simulink library "MyPMSMLibrary"  (R2025b)
settings: Solver=VariableStepAuto  StartTime=0.0  StopTime=10.0  RelTol=1e-3
settings Model: Creator=jff_1  LastModifiedBy=jff_1
settings ModelReferenceCC: EnableRefExpFcnMdlSchedulingChecks=on
settings RTWCC: GPUComputeCapability=3.5

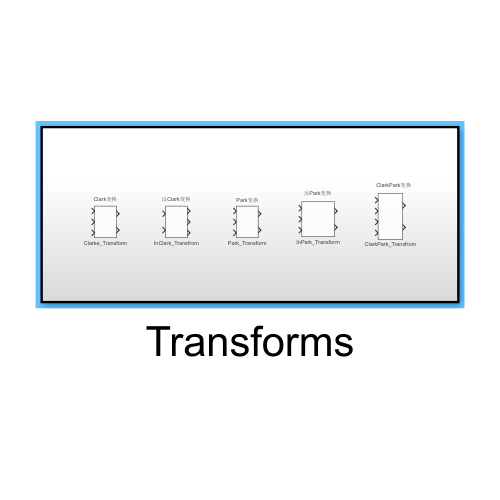
[thumbnail: Simulink's stored preview of the top-level diagram]
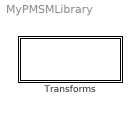
== system MyPMSMLibrary ==
  Transforms : Subsystem

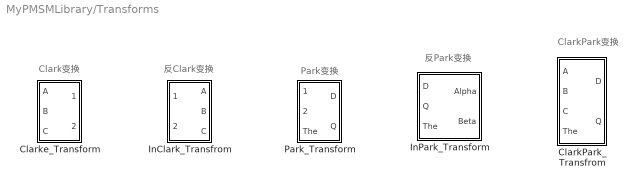
== system MyPMSMLibrary/Transforms ==
  note: 反Clark变换
  note: Clark变换
  note: Park变换
  note: 反Park变换
  note: ClarkPark变换
  ClarkPark_Transfrom : Subsystem
      mask help:
      | 将三相静止坐标系的 A、B、C 量通过同步旋转角 The(θ) 变换到同步旋转坐标系 d、q。
      | 本模块采用 2/3 幅值不变（amplitude-invariant）系数，常用于电机矢量控制中的电流/电压坐标变换。
      mask Help:
      | 【功能】
      | 把三相静止量 (A,B,C) 变换为同步旋转坐标系的 (d,q)，角度由 The(θ) 提供。
      | 
      | 【输入端口】
      | 
      | A：A 相量（电流/电压等）
      | 
      | B：B 相量
      | 
      | C：C 相量
      | 
      | The：同步旋转角 θ（单位：rad，弧度）
      | 
      | 【输出端口】
      | 
      | D：d 轴分量
      | 
      | Q：q 轴分量
      | 
      | 【计算关系（与模块内部 Fcn 一致）】
      | D = ( Acos(The) + Bcos(The - 2/3pi) + Ccos(The + 2/3pi) ) * 2/3
      | Q = -( Asin(The) + Bsin(The - 2/3pi) + Csin(The + 2/3pi) ) * 2/3
      | 
      | 【说明与注意】
      | 
      | The 必须使用弧度制；若你手里是角度制(°)，请先转换：The = The_deg*pi/180。
      | 
      | 该实现等价于“Clarke(abc→αβ) + Park(αβ→dq)”的组合写法，只是把两步合成到一起。
      | 
      | 若输入三相为对称系统（A+B+C=0），该变换结果最稳定；若含零序分量，本模块未单独输出零序。
      | 
      | 【快速自检建议】
      | 
      | 令 The = 0：此时 D 与 A 的相关性最大，Q 主要由 B/C 组合决定。
      | 
      | 令三相为对称正弦并随 The 同步旋转：理想情况下 d 为常值、q 约为 0（或相反，取决于相位定义）。
      mask DialogControl ParameterGroupVar Prompt: 参数
      mask Display:
      | % 输入端口
      | port_label('input',1,'A');
      | port_label('input',2,'B');
      | port_label('input',3,'C');
      | port_label('input',4,'The');
      | 
      | % 输出端口
      | port_label('output',1,'D');
      | port_label('output',2,'Q');
  Clarke_Transform : Subsystem
      mask help:
      | Clarke 坐标变换（abc → αβ）
      |
      | 采用幅值不变形式（2/3 系数）
      | 适用于三相对称、无零序分量的系统
      mask Help: 现代永磁同步电机控制原理及MATLAB仿真P5
      mask DialogControl ParameterGroupVar Prompt: 参数
      mask Display:
      | % 输入端口标签（1~3）
      | port_label('input',1,'A');
      | port_label('input',2,'B');
      | port_label('input',3,'C');
      | 
      | % 输出端口标签（1~2）
      | port_label('output',1,'Alpha');
      | port_label('output',2,'Beta');
  InClark_Transfrom : Subsystem
      mask help:
      | 反Clark坐标变换（αβ → abc）
      |
      | 采用幅值不变形式（2/3 系数）
      | 适用于三相对称、无零序分量的系统
      mask Help: 现代永磁同步电机控制原理及MATLAB仿真P6
      mask DialogControl ParameterGroupVar Prompt: 参数
      mask Display:
      | % 输入端口标签（1~3）
      | port_label('input',1,'Alpha');
      | port_label('input',2,'Beta');
      | 
      | % 输出端口标签（1~2）
      | port_label('output',1,'A');
      | port_label('output',2,'B');
      | port_label('output',3,'C');
  InPark_Transform : Subsystem
      mask help:
      | 反 Park 变换用于将同步旋转坐标系 d–q 中的变量变换回静止坐标系 α–β。
      | 该变换是 Park 变换的逆过程，广泛应用于 PMSM 矢量控制（FOC）中，
      | 用于将 dq 坐标系下的电流或电压还原为 αβ 坐标系量，以便后续调制或坐标变换。
      mask Help:
      | 反 Park 变换的数学表达式为：
      | 
      | [ alpha ]   [ cos(θe)  -sin(θe) ] [ d ]
      | [ beta  ] = [ sin(θe)   cos(θe) ] [ q ]
      | 
      | 即：
      | alpha = d*cos(θe) - q*sin(θe)
      | beta  = d*sin(θe) + q*cos(θe)
      | 
      | 输入端口：
      | D   —— d 轴分量
      | Q   —— q 轴分量
      | The —— 同步旋转角 θe（rad）
      | 
      | 输出端口：
      | Alpha —— α 轴分量
      | Beta  —— β 轴分量
      | 
      | 本模块通常与 Park 变换模块配合使用，
      | 用于 PMSM 矢量控制中 dq → αβ 的坐标变换。
      mask DialogControl ParameterGroupVar Prompt: 参数
      mask Display:
      | % 输入端口标签
      | port_label('input',1,'D');
      | port_label('input',2,'Q');
      | port_label('input',3,'The');
      | 
      | % 输出端口标签
      | port_label('output',1,'Alpha');
      | port_label('output',2,'Beta');
  Park_Transform : Subsystem
      mask help:
      | Park 变换用于将静止 α-β 坐标系中的物理量转换到同步旋转 d-q 坐标系。
      |
      | 通过引入同步旋转角 θ（通常为电角度），将 α-β 平面上的矢量
      | 旋转到以转子磁场为参考的 d-q 坐标系中，使交流量在稳态下
      | 转化为直流量，便于控制器设计与分析。
      |
      | 该变换广泛应用于永磁同步电机（PMSM）和异步电机的矢量控制中，
      | 是磁场定向控制（FOC）的核心坐标变换之一。
      mask Help:
      | 【功能说明】
      | 本模块实现 Park 坐标变换，将 α-β 静止坐标系下的输入量
      | 转换为同步旋转坐标系下的 d-q 分量。
      | 
      | 【数学表达式】
      | 设输入为：
      |   α  —— α 轴分量
      |   β  —— β 轴分量
      |   θ  —— 同步旋转角（电角度，单位：rad）
      | 
      | 则 Park 变换公式为：
      | 
      |   d =  α·cos(θ) + β·sin(θ)
      |   q = -α·sin(θ) + β·cos(θ)
      | 
      | 矩阵形式表示为：
      | 
      |   [ d ] = [  cosθ   sinθ ] [ α ]
      |   [ q ]   [ -sinθ   cosθ ] [ β ]
      | 
      | 【端口说明】
      | 输入端口：
      |   α     —— α 轴分量
      |   β     —— β 轴分量
      |   θ     —— 同步旋转角（rad）
      | 
      | 输出端口：
      |   d     —— d 轴分量
      |   q     —— q 轴分量
      | 
      | 【使用说明】
      | 1. θ 通常由转子位置或积分电角速度获得；
      | 2. 在 PMSM 矢量控制中：
      |    - d 轴通常用于磁链控制
      |    - q 轴通常用于转矩控制
      | 3. 若 α-β 来自 Clarke 变换，则该模块构成完整的
      |    abc → αβ → dq 坐标变换链路。
      | 
      | 【注意事项】
      | - 本模块未包含零序分量；
      | - 输入信号应满足单位一致性（θ 为弧度制）。
      mask DialogControl ParameterGroupVar Prompt: 参数
      mask Display:
      | % 输入端口标签（1~3）
      | port_label('input',1,'Alpha');
      | port_label('input',2,'Beta');
      | port_label('input',3,'The');
      | 
      | % 输出端口标签（1~2）
      | port_label('output',1,'D');
      | port_label('output',2,'Q');

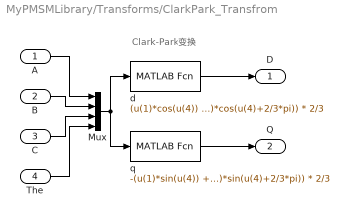
== system MyPMSMLibrary/Transforms/ClarkPark_Transfrom ==
  note: Clark-Park变换
  A : Inport
  B : Inport  Port=2
  C : Inport  Port=3
  The : Inport  Port=4
  Mux : Mux
  d : MATLABFcn  MATLABFcn=(u(1)*cos(u(4)) + u(2)*cos(u(4)-2/3*pi) + u(3)*cos(u(4)+2/3*pi)) * 2/3
  q : MATLABFcn  MATLABFcn=-(u(1)*sin(u(4)) + u(2)*sin(u(4)-2/3*pi) + u(3)*sin(u(4)+2/3*pi)) * 2/3
  D : Outport
  Q : Outport  Port=2
  wires:
  The/1 -> Mux/4
  C/1 -> Mux/3
  B/1 -> Mux/2
  Mux/1 -> q/1, d/1
  q/1 -> Q/1
  d/1 -> D/1
  A/1 -> Mux/1

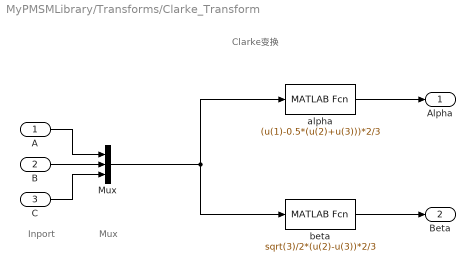
== system MyPMSMLibrary/Transforms/Clarke_Transform ==
  note: Clarke变换
  note: Inport
  note: Mux
  A : Inport
  B : Inport  Port=2
  C : Inport  Port=3
  Mux : Mux  Inputs=3
  alpha : MATLABFcn  MATLABFcn=(u(1)-0.5*(u(2)+u(3)))*2/3
  beta : MATLABFcn  MATLABFcn=sqrt(3)/2*(u(2)-u(3))*2/3
  Alpha : Outport
  Beta : Outport  Port=2
  wires:
  Mux/1 -> beta/1, alpha/1
  beta/1 -> Beta/1
  alpha/1 -> Alpha/1
  C/1 -> Mux/3
  B/1 -> Mux/2
  A/1 -> Mux/1

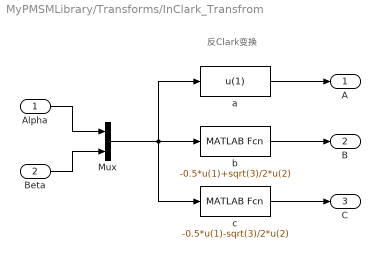
== system MyPMSMLibrary/Transforms/InClark_Transfrom ==
  note: 反Clark变换
  Alpha : Inport
  Beta : Inport  Port=2
  Mux : Mux  Inputs=2
  a : MATLABFcn  MATLABFcn=u(1)
  b : MATLABFcn  MATLABFcn=-0.5*u(1)+sqrt(3)/2*u(2)
  c : MATLABFcn  MATLABFcn=-0.5*u(1)-sqrt(3)/2*u(2)
  A : Outport
  B : Outport  Port=2
  C : Outport  Port=3
  wires:
  Beta/1 -> Mux/2
  a/1 -> A/1
  c/1 -> C/1
  Mux/1 -> c/1, b/1, a/1
  b/1 -> B/1
  Alpha/1 -> Mux/1

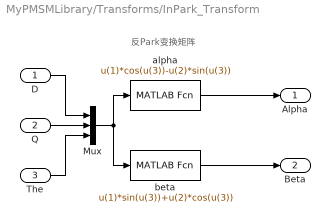
== system MyPMSMLibrary/Transforms/InPark_Transform ==
  note: 反Park变换矩阵
  D : Inport
  Q : Inport  Port=2
  The : Inport  Port=3
  Mux : Mux  Inputs=3
  alpha : MATLABFcn  MATLABFcn=u(1)*cos(u(3))-u(2)*sin(u(3))
  beta : MATLABFcn  MATLABFcn=u(1)*sin(u(3))+u(2)*cos(u(3))
  Alpha : Outport
  Beta : Outport  Port=2
  wires:
  beta/1 -> Beta/1
  The/1 -> Mux/3
  Q/1 -> Mux/2
  Mux/1 -> beta/1, alpha/1
  D/1 -> Mux/1
  alpha/1 -> Alpha/1

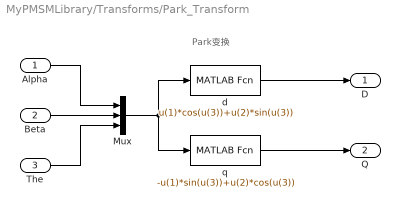
== system MyPMSMLibrary/Transforms/Park_Transform ==
  note: Park变换
  Alpha : Inport
  Beta : Inport  Port=2
  The : Inport  Port=3
  Mux : Mux  Inputs=3
  d : MATLABFcn  MATLABFcn=u(1)*cos(u(3))+u(2)*sin(u(3))
  q : MATLABFcn  MATLABFcn=-u(1)*sin(u(3))+u(2)*cos(u(3))
  D : Outport
  Q : Outport  Port=2
  wires:
  d/1 -> D/1
  The/1 -> Mux/3
  Mux/1 -> q/1, d/1
  q/1 -> Q/1
  Alpha/1 -> Mux/1
  Beta/1 -> Mux/2
